simulink model "FOC"  (R2026a)
settings: Solver=FixedStepDiscrete  StopTime=inf  FixedStep=Ts  EnableMultiTasking=on
InitFcn:
  | ParameterInit
undefined symbols (not defined in the file): drive, FAKF, motor, Ts
libraries: mcbhdlcontrolslib x9, matrix_library x8, simulink x7, mcbcontrolslib x5, mcbsensorlessestimatorlib x2, mcbeeMathTransformLib x2, slpidlib x2, mcbpositiondecoderlib x1, sl_discontinuities x1
(part 2 of 2)

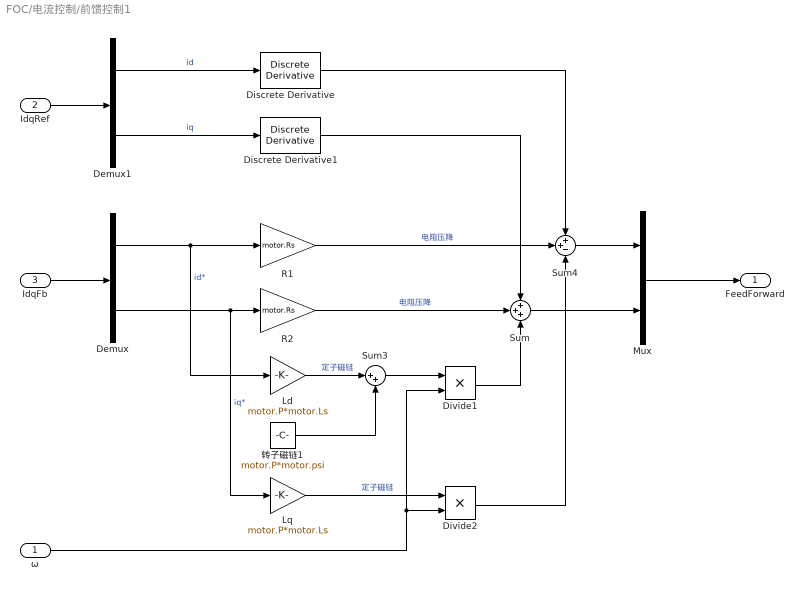
== system FOC/电流控制/前馈控制1 ==
  ω : Inport
  IdqRef : Inport  Port=2
  IdqFb : Inport  Port=3
  Demux : Demux  Outputs=2
  Demux1 : Demux  Outputs=2
  Discrete Derivative : simulink/Discrete/Discrete Derivative  gainval=motor.Ls  ICPrevScaledInput=0.0  OutMin=[]  OutMax=[]  OutDataType=fixdt(1, 16)  OutScaling=2^-10  DoSatur=off
  Discrete Derivative1 : simulink/Discrete/Discrete Derivative  gainval=motor.Ls  ICPrevScaledInput=0.0  OutMin=[]  OutMax=[]  OutDataType=fixdt(1, 16)  OutScaling=2^-10  DoSatur=off
  Divide1 : Product  Inputs=**
  Divide2 : Product  Inputs=**
  Ld : Gain  Gain=motor.P*motor.Ls
  Lq : Gain  Gain=motor.P*motor.Ls
  Mux : Mux  Inputs=2
  R1 : Gain  Gain=motor.Rs
  R2 : Gain  Gain=motor.Rs
  Sum : Sum  Inputs=+++
  Sum3 : Sum  Inputs=|++
  Sum4 : Sum  Inputs=++-
  转子磁链1 : Constant  Value=motor.P*motor.psi  VectorParams1D=off  OutDataTypeStr=single
  FeedForward : Outport
  wires:
  Ld/1 -> Sum3/1  "定子磁链"
  转子磁链1/1 -> Sum3/2
  Lq/1 -> Divide2/1  "定子磁链"
  Sum3/1 -> Divide1/1
  ω/1 -> Divide2/2, Divide1/2
  Demux/1 -> R1/1, Ld/1  "id*"
  Demux/2 -> Lq/1, R2/1  "iq*"
  IdqFb/1 -> Demux/1
  Divide2/1 -> Sum4/3
  Divide1/1 -> Sum/3
  Sum/1 -> Mux/2
  Sum4/1 -> Mux/1
  IdqRef/1 -> Demux1/1
  Demux1/2 -> Discrete Derivative1/1  "iq"
  R2/1 -> Sum/2  "电阻压降"
  R1/1 -> Sum4/2  "电阻压降"
  Discrete Derivative1/1 -> Sum/1
  Discrete Derivative/1 -> Sum4/1
  Mux/1 -> FeedForward/1
  Demux1/1 -> Discrete Derivative/1  "id"

== system FOC/电流控制/电压限幅 ==
  dq_in : Inport
  Limit : Inport  Port=2
  Divide1 : Product  Inputs=*/*
  Math Function1 : Math  Operator=square
  Relational Operator : RelationalOperator  Operator=>  OutDataTypeStr=boolean  RndMeth=Simplest  InputSameDT=off
  Sqrt : Sqrt
  Sum of Elements1 : Sum  Inputs=+
  Switch : Switch  Criteria=u2 > Threshold  SaturateOnIntegerOverflow=off  InputSameDT=off
  dq_out : Outport
  wires:
  Divide1/1 -> Switch/1
  Relational Operator/1 -> Switch/2
  Math Function1/1 -> Sum of Elements1/1
  Switch/1 -> dq_out/1
  Sum of Elements1/1 -> Sqrt/1
  Sqrt/1 -> Relational Operator/1, Divide1/2
  Limit/1 -> Relational Operator/2, Divide1/1
  dq_in/1 -> Divide1/3, Switch/3, Math Function1/1

== system FOC/电流控制/非线性补偿 ==
  U_dq : Inport
  Gain1 : Gain  Gain=[1/(motor.Rs+motor.Ls/Ts) 1/(motor.Rs+motor.Ls/Ts)]
  I_dq : Outport
  wires:
  U_dq/1 -> Gain1/1
  Gain1/1 -> I_dq/1

== system FOC/Observer/AKF/协方差估计 ==
  e~ : Inport
  e^ : Inport  Port=2
  S : Inport  Port=3
  T : Inport  Port=4
  Display : Display
  Display1 : Display
  Unit Delay1 : UnitDelay  InitialCondition=eye(2)  SampleTime=-1
  Unit Delay2 : UnitDelay  InitialCondition=eye(2)  SampleTime=-1
  乘法积分器 : Subsystem
  乘法积分器1 : Subsystem
  息差估计 : Subsystem
  残差估计 : Subsystem
  R : Outport
  Q : Outport  Port=2
  wires:
  Unit Delay2/1 -> 乘法积分器1/2(T)
  T/1 -> Unit Delay2/1
  乘法积分器/1(Q) -> Q/1, Display/1
  乘法积分器1/1(R) -> R/1, Display1/1
  Unit Delay1/1 -> 乘法积分器/2(S)
  息差估计/1(cov) -> 乘法积分器1/1(T~)
  S/1 -> Unit Delay1/1
  e^/1 -> 残差估计/1(ωθ)
  残差估计/1(cov) -> 乘法积分器/1(S~)
  e~/1 -> 息差估计/1(ωθ)

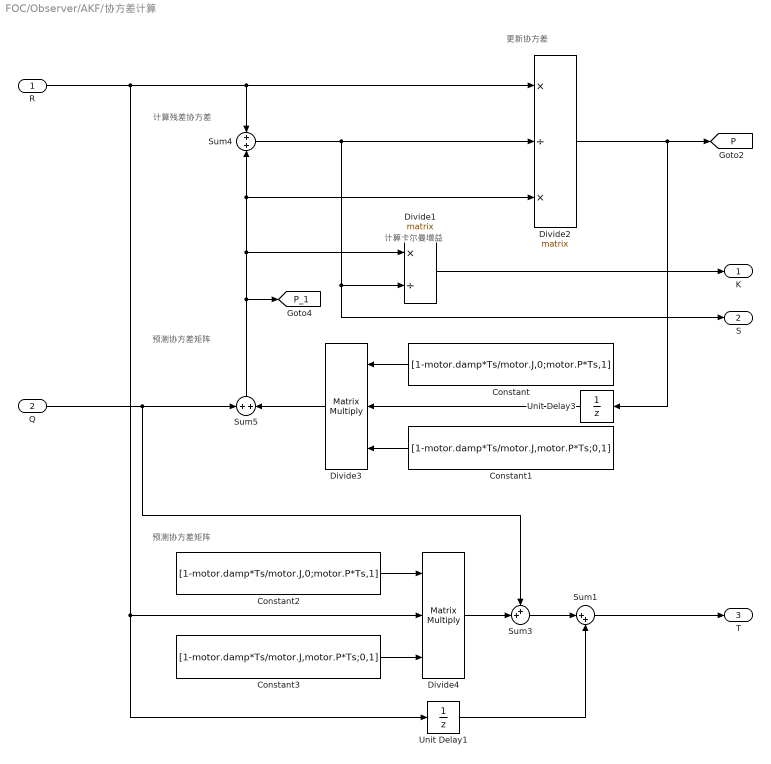
== system FOC/Observer/AKF/协方差计算 ==
  note: 预测协方差矩阵
  note: 更新协方差
  note: 计算卡尔曼增益
  note: 计算残差协方差
  note: 预测协方差矩阵
  R : Inport
  Q : Inport  Port=2
  Constant : Constant  Value=[1-motor.damp*Ts/motor.J,0;motor.P*Ts,1]  VectorParams1D=off  OutDataTypeStr=single
  Constant1 : Constant  Value=[1-motor.damp*Ts/motor.J,motor.P*Ts;0,1]  VectorParams1D=off  OutDataTypeStr=single
  Constant2 : Constant  Value=[1-motor.damp*Ts/motor.J,0;motor.P*Ts,1]  VectorParams1D=off  OutDataTypeStr=single
  Constant3 : Constant  Value=[1-motor.damp*Ts/motor.J,motor.P*Ts;0,1]  VectorParams1D=off  OutDataTypeStr=single
  Divide1 : Product  Inputs=*/  Multiplication=Matrix(*)
  Divide2 : Product  Inputs=*/*  Multiplication=Matrix(*)
  Divide3 : Product  Inputs=***  Multiplication=Matrix(*)
  Divide4 : Product  Inputs=***  Multiplication=Matrix(*)
  Sum1 : Sum  Inputs=|++
  Sum3 : Sum  Inputs=++|
  Sum4 : Sum  Inputs=+|+
  Sum5 : Sum  Inputs=+|+
  Unit Delay1 : UnitDelay  InitialCondition=eye(2)  SampleTime=-1
  Unit Delay3 : UnitDelay  InitialCondition=eye(2)  SampleTime=-1
  K : Outport
  S : Outport  Port=2
  T : Outport  Port=3
  tag scope: P=global, P_1=global
  wires:
  Q/1 -> Sum5/1, Sum3/1
  Unit Delay1/1 -> Sum1/2
  Sum1/1 -> T/1
  R/1 -> Sum4/1, Divide2/1, Divide4/2, Unit Delay1/1
  Sum3/1 -> Sum1/1
  Divide4/1 -> Sum3/2
  Constant2/1 -> Divide4/1
  Constant3/1 -> Divide4/3
  Divide1/1 -> K/1
  Sum4/1 -> Divide2/2, Divide1/2, S/1
  Unit Delay3/1 -> Divide3/2
  Constant1/1 -> Divide3/3
  Divide3/1 -> Sum5/2
  Divide2/1 -> Unit Delay3/1, [P]
  Constant/1 -> Divide3/1
  Sum5/1 -> Sum4/2, Divide2/3, Divide1/1, [P_1]

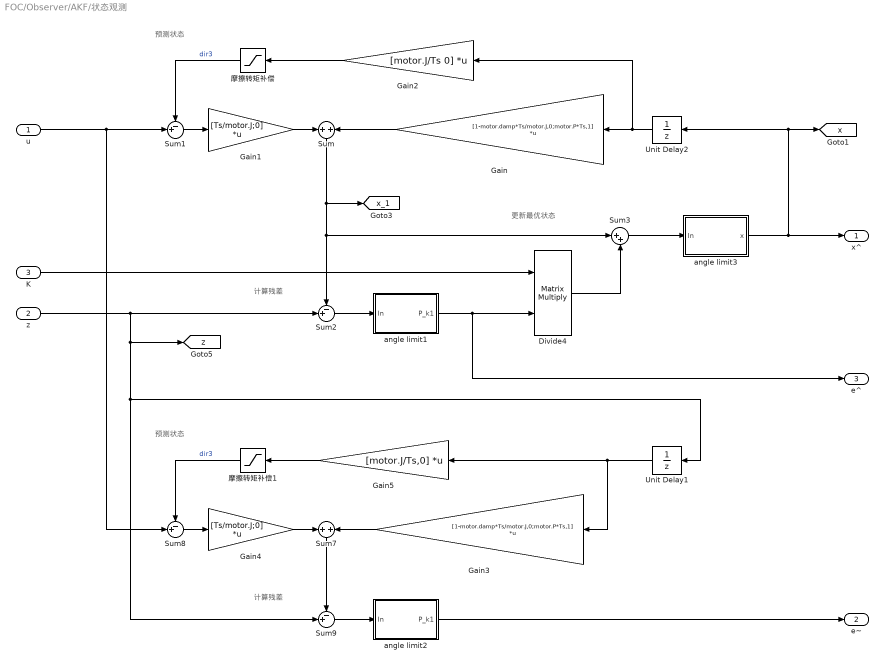
== system FOC/Observer/AKF/状态观测 ==
  note: 计算残差
  note: 预测状态
  note: 更新最优状态
  note: 计算残差
  note: 预测状态
  u : Inport
  z : Inport  Port=2
  K : Inport  Port=3
  Divide4 : Product  Inputs=**  Multiplication=Matrix(*)
  Gain : Gain  Gain=[1-motor.damp*Ts/motor.J,0;motor.P*Ts,1]  Multiplication=Matrix(K*u)
  Gain1 : Gain  Gain=[Ts/motor.J;0]  Multiplication=Matrix(K*u)
  Gain2 : Gain  Gain=[motor.J/Ts 0]  Multiplication=Matrix(K*u)
  Gain3 : Gain  Gain=[1-motor.damp*Ts/motor.J,0;motor.P*Ts,1]  Multiplication=Matrix(K*u)
  Gain4 : Gain  Gain=[Ts/motor.J;0]  Multiplication=Matrix(K*u)
  Gain5 : Gain  Gain=[motor.J/Ts,0]  Multiplication=Matrix(K*u)
  Sum : Sum  Inputs=+|+
  Sum{1..2,8..9} (4 alike) : Sum  Inputs=-+|
  Sum3 : Sum  Inputs=|++
  Sum7 : Sum  Inputs=+|+
  Unit Delay1 : UnitDelay  SampleTime=-1
  Unit Delay2 : UnitDelay  SampleTime=-1
  angle limit1 : Subsystem
  angle limit2 : Subsystem
  angle limit3 : Subsystem
  摩擦转矩补偿 : Saturate  UpperLimit=motor.fric  LowerLimit=-motor.fric
  摩擦转矩补偿1 : Saturate  UpperLimit=motor.fric  LowerLimit=-motor.fric
  x^ : Outport
  e~ : Outport  Port=2
  e^ : Outport  Port=3
  tag scope: x=global, x_1=global, z=global
  wires:
  摩擦转矩补偿/1 -> Sum1/1  "dir3"
  摩擦转矩补偿1/1 -> Sum8/1  "dir3"
  angle limit2/1(P_k1) -> e~/1
  K/1 -> Divide4/1
  z/1 -> Unit Delay1/1, Sum9/2, [z], Sum2/2
  u/1 -> Sum8/2, Sum1/2
  Unit Delay1/1 -> Gain5/1, Gain3/1
  Sum8/1 -> Gain4/1
  Sum2/1 -> angle limit1/1(In)
  Sum9/1 -> angle limit2/1(In)
  angle limit3/1(x) -> Unit Delay2/1, [x], x^/1
  Sum7/1 -> Sum9/1
  Gain2/1 -> 摩擦转矩补偿/1
  Sum1/1 -> Gain1/1
  Divide4/1 -> Sum3/2
  Unit Delay2/1 -> Gain/1, Gain2/1
  Gain5/1 -> 摩擦转矩补偿1/1
  Gain3/1 -> Sum7/2
  Gain/1 -> Sum/2
  Gain1/1 -> Sum/1
  Gain4/1 -> Sum7/1
  Sum3/1 -> angle limit3/1(In)
  angle limit1/1(P_k1) -> Divide4/2, e^/1
  Sum/1 -> Sum3/1, Sum2/1, [x_1]

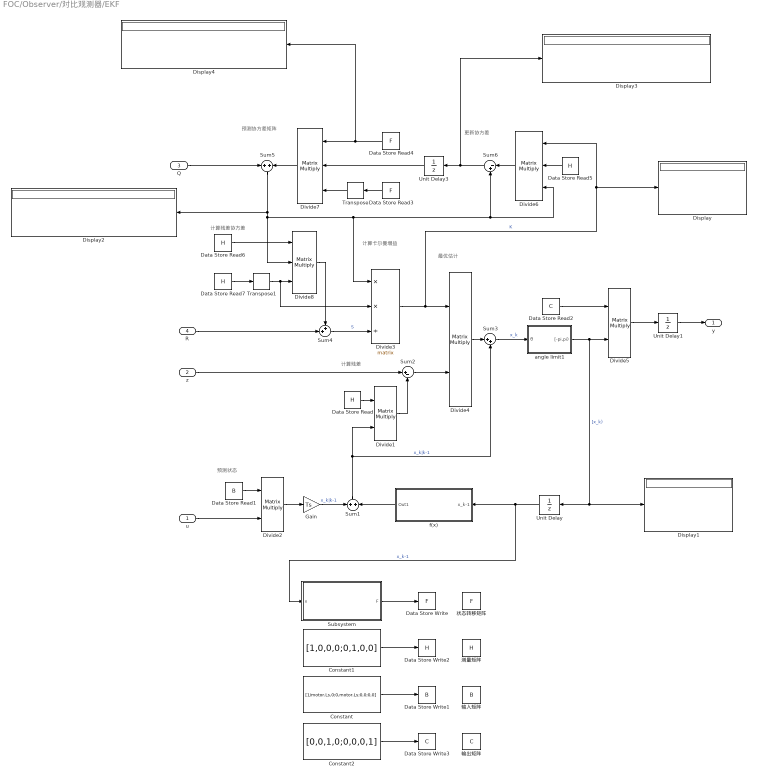
== system FOC/Observer/对比观测器/EKF ==
  note: 更新协方差
  note: 计算卡尔曼增益
  note: 预测协方差矩阵
  note: 计算残差协方差
  note: 最优估计
  note: 计算残差
  note: 预测状态
  u : Inport
  z : Inport  Port=2
  Q : Inport  Port=3
  R : Inport  Port=4
  Constant : Constant  Value=[1/motor.Ls,0;0,motor.Ls;0,0;0,0]  VectorParams1D=off  OutDataTypeStr=single
  Constant1 : Constant  Value=[1,0,0,0;0,1,0,0]  VectorParams1D=off  OutDataTypeStr=single
  Constant2 : Constant  Value=[0,0,1,0;0,0,0,1]  VectorParams1D=off  OutDataTypeStr=single
  Data Store Read{,5..7} (4 alike) : DataStoreRead  DataStoreName=H  IndexOptions=Index vector (dialog)  Indices=1  OutputSizes=1
  Data Store Read1 : DataStoreRead  DataStoreName=B  IndexOptions=Index vector (dialog)  Indices=1  OutputSizes=1
  Data Store Read2 : DataStoreRead  DataStoreName=C  IndexOptions=Index vector (dialog)  Indices=1  OutputSizes=1
  Data Store Read3 : DataStoreRead  DataStoreName=F  IndexOptions=Index vector (dialog)  Indices=1  OutputSizes=1
  Data Store Read4 : DataStoreRead  DataStoreName=F  IndexOptions=Index vector (dialog)  Indices=1  OutputSizes=1
  Data Store Write : DataStoreWrite  DataStoreName=F  IndexOptions=Index vector (dialog)  Indices=1  OutputSizes=1
  Data Store Write1 : DataStoreWrite  DataStoreName=B  IndexOptions=Index vector (dialog)  Indices=1  OutputSizes=1
  Data Store Write2 : DataStoreWrite  DataStoreName=H  IndexOptions=Index vector (dialog)  Indices=1  OutputSizes=1
  Data Store Write3 : DataStoreWrite  DataStoreName=C  IndexOptions=Index vector (dialog)  Indices=1  OutputSizes=1
  Display{,1..4} (5 alike) : Display
  Divide{1..2,4..5} (4 alike) : Product  Inputs=**  Multiplication=Matrix(*)
  Divide3 : Product  Inputs=**/  Multiplication=Matrix(*)
  Divide6 : Product  Inputs=***  Multiplication=Matrix(*)
  Divide7 : Product  Inputs=***  Multiplication=Matrix(*)
  Divide8 : Product  Inputs=***  Multiplication=Matrix(*)
  Gain : Gain  Gain=Ts
  Subsystem : Subsystem
  Sum1 : Sum  Inputs=+|+
  Sum2 : Sum  Inputs=|+-
  Sum3 : Sum  Inputs=|++
  Sum4 : Sum  Inputs=++|
  Sum5 : Sum  Inputs=+|+
  Sum6 : Sum  Inputs=|-+
  Transpose : matrix_library/Transpose
  Transpose1 : matrix_library/Transpose
  Unit Delay : UnitDelay  InitialCondition=zeros(4,1)  SampleTime=-1
  Unit Delay1 : UnitDelay  InitialCondition=zeros(2,1)  SampleTime=-1
  Unit Delay3 : UnitDelay  InitialCondition=diag([1e0,1e0,1000*[1,Ts^2/4]])  SampleTime=-1
  angle limit1 : Subsystem
  f(x) : Subsystem
  测量矩阵 : DataStoreMemory  DataStoreName=H  WriteAfterWriteMsg=warning  InitialValue=[1,0,0,0;0,1,0,0]  VectorParams1D=off  ShowAdditionalParam=off
  状态转移矩阵 : DataStoreMemory  DataStoreName=F  WriteAfterWriteMsg=warning  InitialValue=eye(4)  VectorParams1D=off  ShowAdditionalParam=off
  输入矩阵 : DataStoreMemory  DataStoreName=B  WriteAfterWriteMsg=warning  InitialValue=[1/motor.Ls,0;0,motor.Ls;0,0;0,0]  VectorParams1D=off  ShowAdditionalParam=off
  输出矩阵 : DataStoreMemory  DataStoreName=C  WriteAfterWriteMsg=warning  InitialValue=[0,0,1,0;0,0,0,1]  VectorParams1D=off  ShowAdditionalParam=off
  y : Outport
  wires:
  Data Store Read4/1 -> Divide7/1, Display4/1
  Sum6/1 -> Unit Delay3/1, Display3/1
  Unit Delay1/1 -> y/1
  Divide8/1 -> Sum4/1
  Data Store Read6/1 -> Divide8/1
  Transpose1/1 -> Divide8/3, Divide3/2
  Data Store Read7/1 -> Transpose1/1
  Constant2/1 -> Data Store Write3/1
  Divide1/1 -> Sum2/2
  Data Store Read/1 -> Divide1/1
  Gain/1 -> Sum1/1  "x_k|k-1"
  angle limit1/1("[-pi,pi)") -> Unit Delay/1, Display1/1, Divide5/2  "[x_k)"
  f(x)/1(Out1) -> Sum1/2
  Subsystem/1(F) -> Data Store Write/1
  Transpose/1 -> Divide7/3
  Divide6/1 -> Sum6/1
  Data Store Read5/1 -> Divide6/2
  Data Store Read3/1 -> Transpose/1
  Sum4/1 -> Divide3/3  "S"
  Unit Delay3/1 -> Divide7/2
  R/1 -> Sum4/2
  Divide7/1 -> Sum5/2
  Sum5/1 -> Display2/1, Divide8/2, Sum6/2, Divide6/3, Divide3/1
  Q/1 -> Sum5/1
  Constant1/1 -> Data Store Write2/1
  Constant/1 -> Data Store Write1/1
  Divide5/1 -> Unit Delay1/1
  Data Store Read1/1 -> Divide2/1
  z/1 -> Sum2/1
  Sum2/1 -> Divide4/2
  Divide4/1 -> Sum3/1
  Divide2/1 -> Gain/1
  Unit Delay/1 -> f(x)/1(x_k-1), Subsystem/1(x)  "x_k-1"
  Data Store Read2/1 -> Divide5/1
  u/1 -> Divide2/2
  Sum1/1 -> Sum3/2, Divide1/2  "x_k|k-1"
  Divide3/1 -> Divide4/1, Divide6/1, Display/1  "K"
  Sum3/1 -> angle limit1/1(θ)  "x_k"

== system FOC/Observer/对比观测器/FKF ==
  z : Inport
  u : Inport  Port=2
  AKF : Subsystem
  Demux : Demux  Outputs=2
  位置提取 : Subsystem
  角度转换 : Subsystem
  计算转子反电动势 : Subsystem
  转矩计算 : Subsystem
  ω_m : Outport
  θ_e : Outport  Port=2
  wires:
  位置提取/1(ωθ) -> AKF/2(z_k)  "ωθ~"
  角度转换/1(sincos) -> 位置提取/2(θ_sincos), 转矩计算/1(θ_sincos)
  AKF/1(x_k) -> Demux/1
  u/1 -> 计算转子反电动势/2(Uαβ)
  Demux/1 -> ω_m/1
  Demux/2 -> 角度转换/1(θ), θ_e/1
  计算转子反电动势/1(Eαβ) -> 位置提取/1(Eαβ)  "E_αβ"
  z/1 -> 转矩计算/2(I_αβ), 计算转子反电动势/1(Iαβ)
  转矩计算/1(T) -> AKF/1(u_k)  "T"

== system FOC/Observer/对比观测器/Subsystem ==
  θ_e : Inport
  Constant2 : Constant  Value=-pi  OutDataTypeStr=single
  Constant4 : Constant  Value=pi  OutDataTypeStr=single
  Difference : simulink/Discrete/Difference  ICPrevInput=0.0  OutMin=[]  OutMax=[]  OutDataType=fixdt(1, 16)  OutScaling=2^-10  DoSatur=off
  Gain : Gain  Gain=1/(motor.P*Ts)
  Gain6 : Gain  Gain=-2*pi  OutDataTypeStr=single
  Gain7 : Gain  Gain=2*pi  OutDataTypeStr=single
  Relational Operator2 : RelationalOperator  Operator=<  RndMeth=Simplest  InputSameDT=off
  Relational Operator3 : RelationalOperator  Operator=<=  RndMeth=Simplest  InputSameDT=off
  Sum3 : Sum  Inputs=+++
  Y : Outport
  wires:
  Gain/1 -> Y/1
  Constant2/1 -> Relational Operator2/2
  Relational Operator3/1 -> Gain6/1
  Gain7/1 -> Sum3/3
  Constant4/1 -> Relational Operator3/1
  Relational Operator2/1 -> Gain7/1
  Gain6/1 -> Sum3/1
  Difference/1 -> Relational Operator3/2, Sum3/2, Relational Operator2/1
  Sum3/1 -> Gain/1
  θ_e/1 -> Difference/1

== system FOC/Observer/对比观测器/Subsystem1 ==
  0-2pi : Inport
  Constant3 : Constant  Value=-pi  OutDataTypeStr=single
  Constant4 : Constant  Value=pi  OutDataTypeStr=single
  Gain6 : Gain  Gain=-2*pi  OutDataTypeStr=single
  Gain7 : Gain  Gain=2*pi  OutDataTypeStr=single
  Relational Operator2 : RelationalOperator  Operator=<  RndMeth=Simplest  InputSameDT=off
  Relational Operator3 : RelationalOperator  Operator=<  RndMeth=Simplest  InputSameDT=off
  Sum3 : Sum  Inputs=+++
  -pi-pi : Outport
  wires:
  Sum3/1 -> -pi-pi/1
  Gain7/1 -> Sum3/3
  Gain6/1 -> Sum3/1
  Relational Operator3/1 -> Gain6/1
  Relational Operator2/1 -> Gain7/1
  0-2pi/1 -> Relational Operator3/2, Sum3/2, Relational Operator2/1
  Constant3/1 -> Relational Operator2/2
  Constant4/1 -> Relational Operator3/1

== system FOC/Observer/对比观测器/Subsystem2 ==
  0-2pi : Inport
  Constant3 : Constant  Value=-pi  OutDataTypeStr=single
  Constant4 : Constant  Value=pi  OutDataTypeStr=single
  Gain6 : Gain  Gain=-2*pi  OutDataTypeStr=single
  Gain7 : Gain  Gain=2*pi  OutDataTypeStr=single
  Relational Operator2 : RelationalOperator  Operator=<  RndMeth=Simplest  InputSameDT=off
  Relational Operator3 : RelationalOperator  Operator=<  RndMeth=Simplest  InputSameDT=off
  Sum3 : Sum  Inputs=+++
  -pi-pi : Outport
  wires:
  Constant4/1 -> Relational Operator3/1
  Constant3/1 -> Relational Operator2/2
  0-2pi/1 -> Relational Operator2/1, Sum3/2, Relational Operator3/2
  Relational Operator2/1 -> Gain7/1
  Relational Operator3/1 -> Gain6/1
  Gain6/1 -> Sum3/1
  Gain7/1 -> Sum3/3
  Sum3/1 -> -pi-pi/1

== system FOC/Observer/对比观测器/Subsystem3 ==
  0-2pi : Inport
  Constant3 : Constant  Value=-pi  OutDataTypeStr=single
  Constant4 : Constant  Value=pi  OutDataTypeStr=single
  Gain6 : Gain  Gain=-2*pi  OutDataTypeStr=single
  Gain7 : Gain  Gain=2*pi  OutDataTypeStr=single
  Relational Operator2 : RelationalOperator  Operator=<  RndMeth=Simplest  InputSameDT=off
  Relational Operator3 : RelationalOperator  Operator=<  RndMeth=Simplest  InputSameDT=off
  Sum3 : Sum  Inputs=+++
  -pi-pi : Outport
  wires:
  Sum3/1 -> -pi-pi/1
  Gain7/1 -> Sum3/3
  Gain6/1 -> Sum3/1
  Relational Operator3/1 -> Gain6/1
  Relational Operator2/1 -> Gain7/1
  0-2pi/1 -> Relational Operator3/2, Sum3/2, Relational Operator2/1
  Constant3/1 -> Relational Operator2/2
  Constant4/1 -> Relational Operator3/1

== system FOC/Observer/AKF/协方差估计/乘法积分器 ==
  note: 矩阵指数运算量比较大，用一阶泰勒展开式近似
  S~ : Inport
  S : Inport  Port=2
  Divide1 : Product  Inputs=*/  Multiplication=Matrix(*)
  Divide2 : Product  Inputs=***  Multiplication=Matrix(*)
  Gain1 : Gain  Gain=FAKF.fg
  Gain2 : Gain  Gain=1-FAKF.fg
  Sum3 : Sum  Inputs=|++
  Transpose2 : matrix_library/Transpose
  Unit Delay2 : UnitDelay  InitialCondition=eye(2)  SampleTime=-1
  Q : Outport
  wires:
  S/1 -> Divide1/2
  S~/1 -> Divide1/1
  Sum3/1 -> Q/1, Unit Delay2/1
  Transpose2/1 -> Divide2/3
  Gain1/1 -> Sum3/1
  Divide1/1 -> Transpose2/1, Divide2/1
  Gain2/1 -> Sum3/2
  Divide2/1 -> Gain1/1
  Unit Delay2/1 -> Gain2/1, Divide2/2

== system FOC/Observer/AKF/协方差估计/乘法积分器1 ==
  note: 矩阵指数运算量比较大，用一阶泰勒展开式近似
  T~ : Inport
  T : Inport  Port=2
  Divide1 : Product  Inputs=*/  Multiplication=Matrix(*)
  Divide2 : Product  Inputs=***  Multiplication=Matrix(*)
  Gain1 : Gain  Gain=FAKF.fg
  Gain2 : Gain  Gain=1-FAKF.fg
  Sum3 : Sum  Inputs=|++
  Transpose2 : matrix_library/Transpose
  Unit Delay2 : UnitDelay  InitialCondition=eye(2)  SampleTime=-1
  R : Outport
  wires:
  Unit Delay2/1 -> Divide2/2, Gain2/1
  Divide2/1 -> Gain1/1
  Gain2/1 -> Sum3/2
  Divide1/1 -> Divide2/1, Transpose2/1
  Gain1/1 -> Sum3/1
  Transpose2/1 -> Divide2/3
  Sum3/1 -> Unit Delay2/1, R/1
  T~/1 -> Divide1/1
  T/1 -> Divide1/2

== system FOC/Observer/AKF/协方差估计/息差估计 ==
  ωθ : Inport
  Demux1 : Demux  Outputs=2
  IIR Filter1 : mcbcontrolslib/IIR Filter  VariantControl=Low Pass Filter  VariantSelect=Low-pass  FilterConstantInputType=Specify via dialog  Filter_constant=FAKF.fg  InitialOutput=Specify via dialog  InitialOutputValue=0  ExternalReset=none  advancedSettings=off  Ts=50e-6  cutOff_freq=167.5315
  Matrix Concatenate : Concatenate  Mode=Multidimensional array
  Matrix Concatenate1 : Concatenate  Mode=Multidimensional array
  Matrix Concatenate2 : Concatenate  Mode=Multidimensional array  ConcatenateDimension=2
  Product : Product
  Product1 : Product
  Product3 : Product
  cov : Outport
  wires:
  IIR Filter1/1 -> cov/1
  Demux1/2 -> Product1/2, Product3/1, Product3/2
  ωθ/1 -> Demux1/1
  Product3/1 -> Matrix Concatenate1/2
  Product1/1 -> Matrix Concatenate1/1, Matrix Concatenate/2
  Product/1 -> Matrix Concatenate/1
  Matrix Concatenate/1 -> Matrix Concatenate2/1
  Matrix Concatenate1/1 -> Matrix Concatenate2/2
  Matrix Concatenate2/1 -> IIR Filter1/1
  Demux1/1 -> Product/2, Product/1, Product1/1

== system FOC/Observer/AKF/协方差估计/残差估计 ==
  ωθ : Inport
  Demux1 : Demux  Outputs=2
  Gain : Gain  Gain=Ts/2
  IIR Filter1 : mcbcontrolslib/IIR Filter  VariantControl=Low Pass Filter  VariantSelect=Low-pass  FilterConstantInputType=Specify via dialog  Filter_constant=FAKF.fg  InitialOutput=Specify via dialog  InitialOutputValue=0  ExternalReset=none  advancedSettings=off  Ts=50e-6  cutOff_freq=167.5315
  Matrix Concatenate : Concatenate  Mode=Multidimensional array
  Matrix Concatenate1 : Concatenate  Mode=Multidimensional array
  Matrix Concatenate2 : Concatenate  Mode=Multidimensional array  ConcatenateDimension=2
  Product : Product
  Product1 : Product
  Product3 : Product
  cov : Outport
  wires:
  Demux1/1 -> Product1/1, Product/1, Product/2, Gain/1
  IIR Filter1/1 -> cov/1
  Matrix Concatenate2/1 -> IIR Filter1/1
  Matrix Concatenate1/1 -> Matrix Concatenate2/2
  Matrix Concatenate/1 -> Matrix Concatenate2/1
  Product/1 -> Matrix Concatenate/1
  Product1/1 -> Matrix Concatenate/2, Matrix Concatenate1/1
  Product3/1 -> Matrix Concatenate1/2
  ωθ/1 -> Demux1/1
  Gain/1 -> Product3/1, Product3/2, Product1/2

== system FOC/Observer/AKF/状态观测/angle limit1 ==
  In : Inport
  Constant2 : Constant  Value=-pi  OutDataTypeStr=single
  Constant4 : Constant  Value=pi  OutDataTypeStr=single
  Demux : Demux  Outputs=2
  Gain6 : Gain  Gain=-2*pi  OutDataTypeStr=single
  Gain7 : Gain  Gain=2*pi  OutDataTypeStr=single
  Mux : Mux  Inputs=2
  Relational Operator2 : RelationalOperator  Operator=<  RndMeth=Simplest  InputSameDT=off
  Relational Operator3 : RelationalOperator  Operator=<  RndMeth=Simplest  InputSameDT=off
  Sum3 : Sum  Inputs=+++
  P_k1 : Outport
  wires:
  Constant2/1 -> Relational Operator2/2
  Demux/2 -> Relational Operator3/2, Sum3/2, Relational Operator2/1
  Constant4/1 -> Relational Operator3/1
  Relational Operator3/1 -> Gain6/1
  Gain7/1 -> Sum3/3
  Relational Operator2/1 -> Gain7/1
  Gain6/1 -> Sum3/1
  Sum3/1 -> Mux/2
  In/1 -> Demux/1
  Mux/1 -> P_k1/1
  Demux/1 -> Mux/1

== system FOC/Observer/AKF/状态观测/angle limit2 ==
  In : Inport
  Constant2 : Constant  Value=-pi  OutDataTypeStr=single
  Constant4 : Constant  Value=pi  OutDataTypeStr=single
  Demux : Demux  Outputs=2
  Gain6 : Gain  Gain=-2*pi  OutDataTypeStr=single
  Gain7 : Gain  Gain=2*pi  OutDataTypeStr=single
  Mux : Mux  Inputs=2
  Relational Operator2 : RelationalOperator  Operator=<  RndMeth=Simplest  InputSameDT=off
  Relational Operator3 : RelationalOperator  Operator=<  RndMeth=Simplest  InputSameDT=off
  Sum3 : Sum  Inputs=+++
  P_k1 : Outport
  wires:
  Constant2/1 -> Relational Operator2/2
  Demux/2 -> Relational Operator3/2, Sum3/2, Relational Operator2/1
  Constant4/1 -> Relational Operator3/1
  Relational Operator3/1 -> Gain6/1
  Gain7/1 -> Sum3/3
  Relational Operator2/1 -> Gain7/1
  Gain6/1 -> Sum3/1
  Sum3/1 -> Mux/2
  In/1 -> Demux/1
  Mux/1 -> P_k1/1
  Demux/1 -> Mux/1

== system FOC/Observer/AKF/状态观测/angle limit3 ==
  In : Inport
  Constant2 : Constant  Value=-pi  OutDataTypeStr=single
  Constant4 : Constant  Value=pi  OutDataTypeStr=single
  Demux : Demux  Outputs=2
  Gain6 : Gain  Gain=-2*pi  OutDataTypeStr=single
  Gain7 : Gain  Gain=2*pi  OutDataTypeStr=single
  Mux : Mux  Inputs=2
  Relational Operator2 : RelationalOperator  Operator=<  RndMeth=Simplest  InputSameDT=off
  Relational Operator3 : RelationalOperator  Operator=<  RndMeth=Simplest  InputSameDT=off
  Sum3 : Sum  Inputs=+++
  x : Outport
  wires:
  Demux/1 -> Mux/1
  Mux/1 -> x/1
  In/1 -> Demux/1
  Sum3/1 -> Mux/2
  Gain6/1 -> Sum3/1
  Relational Operator2/1 -> Gain7/1
  Gain7/1 -> Sum3/3
  Relational Operator3/1 -> Gain6/1
  Constant4/1 -> Relational Operator3/1
  Demux/2 -> Relational Operator2/1, Sum3/2, Relational Operator3/2
  Constant2/1 -> Relational Operator2/2

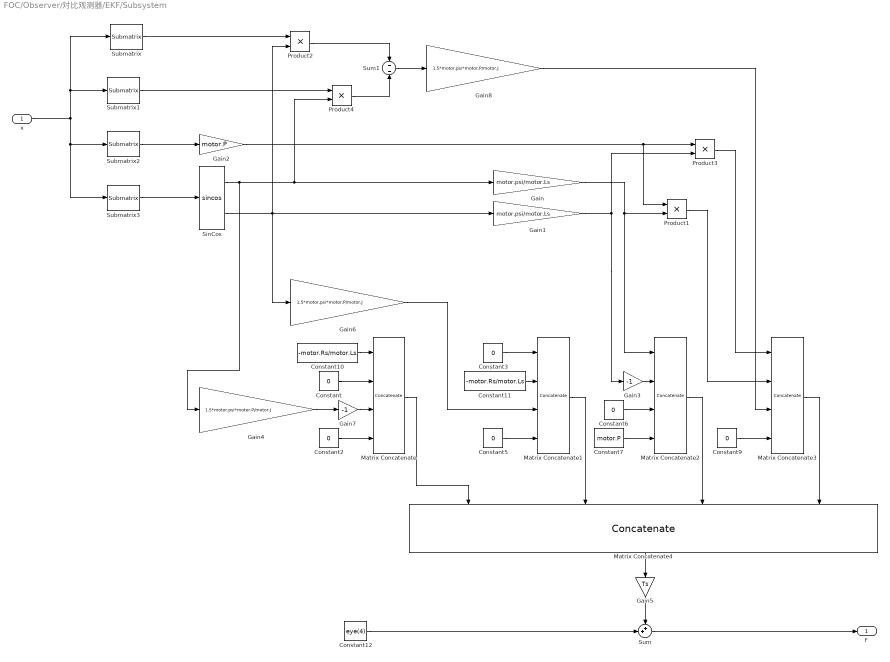
== system FOC/Observer/对比观测器/EKF/Subsystem ==
  x : Inport
  Constant{,2..3,5..6,9} (6 alike) : Constant  Value=0  OutDataTypeStr=single
  Constant10 : Constant  Value=-motor.Rs/motor.Ls  OutDataTypeStr=single
  Constant11 : Constant  Value=-motor.Rs/motor.Ls  OutDataTypeStr=single
  Constant12 : Constant  Value=eye(4)  OutDataTypeStr=single
  Constant7 : Constant  Value=motor.P  OutDataTypeStr=single
  Gain : Gain  Gain=motor.psi/motor.Ls
  Gain1 : Gain  Gain=motor.psi/motor.Ls
  Gain2 : Gain  Gain=motor.P
  Gain3 : Gain  Gain=-1
  Gain4 : Gain  Gain=1.5*motor.psi*motor.P/motor.J
  Gain5 : Gain  Gain=Ts
  Gain6 : Gain  Gain=1.5*motor.psi*motor.P/motor.J
  Gain7 : Gain  Gain=-1
  Gain8 : Gain  Gain=1.5*motor.psi*motor.P/motor.J
  Matrix Concatenate{,1..3} (4 alike) : Concatenate  NumInputs=4  Mode=Multidimensional array
  Matrix Concatenate4 : Concatenate  NumInputs=4  Mode=Multidimensional array  ConcatenateDimension=2
  Product{1..4} (4 alike) : Product
  SinCos : Trigonometry  Operator=sincos
  Submatrix : matrix_library/Submatrix  RowSpan=Range of rows  RowStartMode=Index  RowStartIndex=1  RowEndMode=Index  RowEndIndex=1  ColSpan=One column  ColStartMode=First  ColStartIndex=1  ColEndMode=Index  ColEndIndex=1
  Submatrix1 : matrix_library/Submatrix  RowSpan=Range of rows  RowStartMode=Index  RowStartIndex=2  RowEndMode=Index  RowEndIndex=2  ColSpan=One column  ColStartMode=First  ColStartIndex=1  ColEndMode=Index  ColEndIndex=1
  Submatrix2 : matrix_library/Submatrix  RowSpan=Range of rows  RowStartMode=Index  RowStartIndex=3  RowEndMode=Index  RowEndIndex=3  ColSpan=One column  ColStartMode=First  ColStartIndex=1  ColEndMode=Index  ColEndIndex=1
  Submatrix3 : matrix_library/Submatrix  RowSpan=Range of rows  RowStartMode=Index  RowStartIndex=4  RowEndMode=Index  RowEndIndex=4  ColSpan=One column  ColStartMode=First  ColStartIndex=1  ColEndMode=Index  ColEndIndex=1
  Sum : Sum  Inputs=++|
  Sum1 : Sum  Inputs=-|-
  F : Outport
  wires:
  Sum1/1 -> Gain8/1
  Product4/1 -> Sum1/2
  Product2/1 -> Sum1/1
  Submatrix1/1 -> Product4/1
  Submatrix/1 -> Product2/1
  Gain7/1 -> Matrix Concatenate/3
  Gain3/1 -> Matrix Concatenate2/2
  Gain2/1 -> Product3/1, Product1/1
  Submatrix2/1 -> Gain2/1
  Submatrix3/1 -> SinCos/1
  Gain5/1 -> Sum/1
  Matrix Concatenate4/1 -> Gain5/1
  Constant12/1 -> Sum/2
  Gain1/1 -> Gain3/1, Product3/2
  SinCos/2 -> Gain1/1, Product2/2, Gain6/1
  SinCos/1 -> Gain4/1, Product4/2, Gain/1
  x/1 -> Submatrix/1, Submatrix1/1, Submatrix2/1, Submatrix3/1
  Product1/1 -> Matrix Concatenate3/2
  Product3/1 -> Matrix Concatenate3/1
  Gain/1 -> Product1/2, Matrix Concatenate2/1
  Matrix Concatenate3/1 -> Matrix Concatenate4/4
  Constant9/1 -> Matrix Concatenate3/4
  Constant11/1 -> Matrix Concatenate1/2
  Matrix Concatenate2/1 -> Matrix Concatenate4/3
  Gain4/1 -> Gain7/1
  Matrix Concatenate1/1 -> Matrix Concatenate4/2
  Gain6/1 -> Matrix Concatenate1/3
  Gain8/1 -> Matrix Concatenate3/3
  Constant10/1 -> Matrix Concatenate/1
  Constant6/1 -> Matrix Concatenate2/3
  Sum/1 -> F/1
  Constant7/1 -> Matrix Concatenate2/4
  Matrix Concatenate/1 -> Matrix Concatenate4/1
  Constant5/1 -> Matrix Concatenate1/4
  Constant3/1 -> Matrix Concatenate1/1
  Constant/1 -> Matrix Concatenate/2
  Constant2/1 -> Matrix Concatenate/4

== system FOC/Observer/对比观测器/EKF/angle limit1 ==
  θ : Inport
  Constant2 : Constant  Value=-pi  OutDataTypeStr=single
  Constant4 : Constant  Value=pi  OutDataTypeStr=single
  Demux : Demux
  Gain6 : Gain  Gain=-2*pi  OutDataTypeStr=single
  Gain7 : Gain  Gain=2*pi  OutDataTypeStr=single
  Mux : Mux
  Relational Operator2 : RelationalOperator  Operator=<  RndMeth=Simplest  InputSameDT=off
  Relational Operator3 : RelationalOperator  Operator=<=  RndMeth=Simplest  InputSameDT=off
  Sum3 : Sum  Inputs=+++
  "[-pi,pi)" : Outport
  wires:
  Demux/2 -> Mux/2
  Demux/3 -> Mux/3
  Constant2/1 -> Relational Operator2/2
  Demux/4 -> Relational Operator3/2, Sum3/2, Relational Operator2/1
  Constant4/1 -> Relational Operator3/1
  Relational Operator3/1 -> Gain6/1
  Gain7/1 -> Sum3/3
  Relational Operator2/1 -> Gain7/1
  Gain6/1 -> Sum3/1
  Sum3/1 -> Mux/4
  θ/1 -> Demux/1
  Mux/1 -> "[-pi,pi)"/1
  Demux/1 -> Mux/1

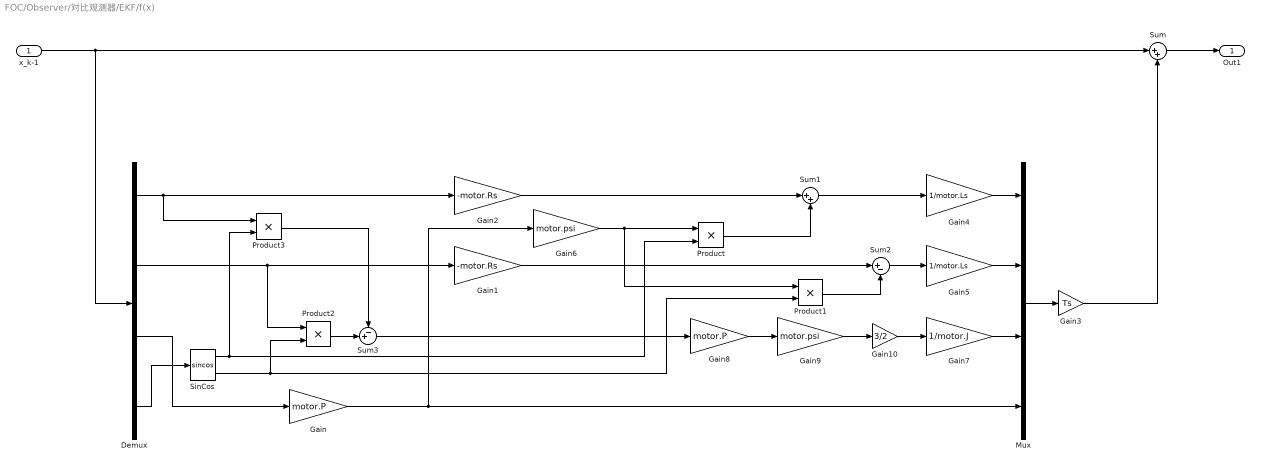
== system FOC/Observer/对比观测器/EKF/f(x) ==
  x_k-1 : Inport
  Demux : Demux
  Gain : Gain  Gain=motor.P
  Gain1 : Gain  Gain=-motor.Rs
  Gain10 : Gain  Gain=3/2
  Gain2 : Gain  Gain=-motor.Rs
  Gain3 : Gain  Gain=Ts
  Gain4 : Gain  Gain=1/motor.Ls
  Gain5 : Gain  Gain=1/motor.Ls
  Gain6 : Gain  Gain=motor.psi
  Gain7 : Gain  Gain=1/motor.J
  Gain8 : Gain  Gain=motor.P
  Gain9 : Gain  Gain=motor.psi
  Mux : Mux
  Product{,1..3} (4 alike) : Product
  SinCos : Trigonometry  Operator=sincos
  Sum : Sum  Inputs=|++
  Sum1 : Sum  Inputs=|++
  Sum2 : Sum  Inputs=|+-
  Sum3 : Sum  Inputs=-+|
  Out1 : Outport
  wires:
  Sum3/1 -> Gain8/1
  Product3/1 -> Sum3/1
  Product2/1 -> Sum3/2
  Gain9/1 -> Gain10/1
  Gain10/1 -> Gain7/1
  Gain8/1 -> Gain9/1
  SinCos/2 -> Product2/2, Product1/2
  Product1/1 -> Sum2/2
  SinCos/1 -> Product3/2, Product/2
  Gain6/1 -> Product/1, Product1/1
  Product/1 -> Sum1/2
  Gain/1 -> Mux/4, Gain6/1
  Sum/1 -> Out1/1
  Demux/3 -> Gain/1
  Gain7/1 -> Mux/3
  Demux/4 -> SinCos/1
  Gain5/1 -> Mux/2
  Gain4/1 -> Mux/1
  Gain3/1 -> Sum/2
  Sum2/1 -> Gain5/1
  Sum1/1 -> Gain4/1
  Gain1/1 -> Sum2/1
  Demux/2 -> Product2/1, Gain1/1
  Gain2/1 -> Sum1/1
  Demux/1 -> Product3/1, Gain2/1
  Mux/1 -> Gain3/1
  x_k-1/1 -> Sum/1, Demux/1

== system FOC/Observer/对比观测器/FKF/AKF ==
  u_k : Inport
  z_k : Inport  Port=2
  Constant1 : Constant  Value=[0.1421,-0.077657;0.0001717,0.002415]  VectorParams1D=off  OutDataTypeStr=single
  Constant4 : Constant  Value=[0.3508,7.253;0.000117,0.0586]  VectorParams1D=off  OutDataTypeStr=single
  状态观测 : Subsystem
  x_k : Outport
  wires:
  Constant4/1 -> 状态观测/3(K)  "K"
  状态观测/1(x^) -> x_k/1  "x^"
  z_k/1 -> 状态观测/2(z)
  u_k/1 -> 状态观测/1(u)

== system FOC/Observer/对比观测器/FKF/位置提取 ==
  Eαβ : Inport
  θ_sincos : Inport  Port=2
  Constant : Constant  Value=motor.psi  OutDataTypeStr=single
  Demux : Demux  Outputs=2
  Divide3 : Product  Inputs=/*
  Gain : Gain  Gain=[-1 1]  Multiplication=Matrix(K*u)
  Gain1 : Gain  Gain=motor.P
  Gain2 : Gain  Gain=-1
  Mux : Mux  Inputs=2
  Product : Product
  Product1 : Product
  Sign : Signum
  Unit Delay : UnitDelay  SampleTime=-1
  幅角 : mcbcontrolslib/atan2  ApproximationMethod=None  NumberOfIterations=11  NumberOfDataPoints=16  InterpMethod=Flat  outputUnit=Radians  TableDataTypeStr=Inherit: Inherit via input
  ωθ : Outport
  wires:
  Product1/1 -> Demux/1
  Sign/1 -> Product1/1
  Eαβ/1 -> Product1/2, Product/2
  Gain2/1 -> 幅角/1
  Demux/1 -> Gain2/1
  Demux/2 -> 幅角/2
  Mux/1 -> ωθ/1
  Divide3/1 -> Mux/1
  Gain/1 -> Sign/1, Divide3/2
  Product/1 -> Gain/1
  Unit Delay/1 -> Product/1
  θ_sincos/1 -> Unit Delay/1
  幅角/1 -> Mux/2
  Gain1/1 -> Divide3/1
  Constant/1 -> Gain1/1

== system FOC/Observer/对比观测器/FKF/角度转换 ==
  θ : Inport
  Mux1 : Mux  Inputs=2
  SinCos : Trigonometry  Operator=sincos
  sincos : Outport
  wires:
  Mux1/1 -> sincos/1
  SinCos/2 -> Mux1/2
  θ/1 -> SinCos/1
  SinCos/1 -> Mux1/1

== system FOC/Observer/对比观测器/FKF/计算转子反电动势 ==
  Iαβ : Inport
  Uαβ : Inport  Port=2
  Sum5 : Sum  Inputs=+--
  滞后补偿 : DiscreteFilter  Numerator=[0 0 1 1]  Denominator=[2 0 0 0]
  电感分压 : simulink/Discrete/Discrete Derivative  gainval=motor.Ls  ICPrevScaledInput=0.0  OutMin=[]  OutMax=[]  OutDataType=fixdt(1, 16)  OutScaling=2^-10  DoSatur=off
  电阻分压 : Gain  Gain=motor.Rs
  Eαβ : Outport
  wires:
  Sum5/1 -> Eαβ/1
  滞后补偿/1 -> Sum5/1
  Iαβ/1 -> 电阻分压/1, 电感分压/1
  Uαβ/1 -> 滞后补偿/1
  电阻分压/1 -> Sum5/2
  电感分压/1 -> Sum5/3

== system FOC/Observer/对比观测器/FKF/转矩计算 ==
  θ_sincos : Inport
  I_αβ : Inport  Port=2
  Constant : Constant  Value=motor.psi  OutDataTypeStr=single
  Divide1 : Product  Inputs=**
  Gain : Gain  Gain=[-1 1]  Multiplication=Matrix(K*u)
  Gain1 : Gain  Gain=motor.P
  Gain2 : Gain  Gain=1.5
  Product3 : Product
  Unit Delay : UnitDelay  SampleTime=-1
  T : Outport
  wires:
  Gain2/1 -> T/1
  Gain1/1 -> Divide1/2
  θ_sincos/1 -> Unit Delay/1
  I_αβ/1 -> Product3/2
  Unit Delay/1 -> Product3/1
  Gain/1 -> Divide1/1
  Divide1/1 -> Gain2/1
  Constant/1 -> Gain1/1
  Product3/1 -> Gain/1

== system FOC/Observer/对比观测器/FKF/AKF/状态观测 ==
  note: 更新最优状态
  note: 计算残差
  note: 预测状态
  u : Inport
  z : Inport  Port=2
  K : Inport  Port=3
  Divide4 : Product  Inputs=**  Multiplication=Matrix(*)
  Gain : Gain  Gain=[1-motor.damp*Ts/motor.J,0;motor.P*Ts,1]  Multiplication=Matrix(K*u)
  Gain1 : Gain  Gain=[Ts/motor.J;0]  Multiplication=Matrix(K*u)
  Gain2 : Gain  Gain=[motor.J/Ts 0]  Multiplication=Matrix(K*u)
  Sum : Sum  Inputs=+|+
  Sum1 : Sum  Inputs=-+|
  Sum2 : Sum  Inputs=-+|
  Sum3 : Sum  Inputs=|++
  Unit Delay2 : UnitDelay  SampleTime=-1
  angle limit1 : Subsystem
  angle limit3 : Subsystem
  摩擦转矩补偿 : Saturate  UpperLimit=motor.fric  LowerLimit=-motor.fric
  x^ : Outport
  wires:
  摩擦转矩补偿/1 -> Sum1/1  "dir3"
  K/1 -> Divide4/1
  z/1 -> Sum2/2
  u/1 -> Sum1/2
  Sum2/1 -> angle limit1/1(In)
  angle limit3/1(x) -> Unit Delay2/1, x^/1
  Gain2/1 -> 摩擦转矩补偿/1
  Sum1/1 -> Gain1/1
  Divide4/1 -> Sum3/2
  Unit Delay2/1 -> Gain/1, Gain2/1
  Gain/1 -> Sum/2
  Gain1/1 -> Sum/1
  Sum3/1 -> angle limit3/1(In)
  angle limit1/1(P_k1) -> Divide4/2
  Sum/1 -> Sum3/1, Sum2/1

== system FOC/Observer/对比观测器/FKF/AKF/状态观测/angle limit1 ==
  In : Inport
  Constant2 : Constant  Value=-pi  OutDataTypeStr=single
  Constant4 : Constant  Value=pi  OutDataTypeStr=single
  Demux : Demux  Outputs=2
  Gain6 : Gain  Gain=-2*pi  OutDataTypeStr=single
  Gain7 : Gain  Gain=2*pi  OutDataTypeStr=single
  Mux : Mux  Inputs=2
  Relational Operator2 : RelationalOperator  Operator=<  RndMeth=Simplest  InputSameDT=off
  Relational Operator3 : RelationalOperator  Operator=<  RndMeth=Simplest  InputSameDT=off
  Sum3 : Sum  Inputs=+++
  P_k1 : Outport
  wires:
  Constant2/1 -> Relational Operator2/2
  Demux/2 -> Relational Operator3/2, Sum3/2, Relational Operator2/1
  Constant4/1 -> Relational Operator3/1
  Relational Operator3/1 -> Gain6/1
  Gain7/1 -> Sum3/3
  Relational Operator2/1 -> Gain7/1
  Gain6/1 -> Sum3/1
  Sum3/1 -> Mux/2
  In/1 -> Demux/1
  Mux/1 -> P_k1/1
  Demux/1 -> Mux/1

== system FOC/Observer/对比观测器/FKF/AKF/状态观测/angle limit3 ==
  In : Inport
  Constant2 : Constant  Value=-pi  OutDataTypeStr=single
  Constant4 : Constant  Value=pi  OutDataTypeStr=single
  Demux : Demux  Outputs=2
  Gain6 : Gain  Gain=-2*pi  OutDataTypeStr=single
  Gain7 : Gain  Gain=2*pi  OutDataTypeStr=single
  Mux : Mux  Inputs=2
  Relational Operator2 : RelationalOperator  Operator=<  RndMeth=Simplest  InputSameDT=off
  Relational Operator3 : RelationalOperator  Operator=<  RndMeth=Simplest  InputSameDT=off
  Sum3 : Sum  Inputs=+++
  x : Outport
  wires:
  Demux/1 -> Mux/1
  Mux/1 -> x/1
  In/1 -> Demux/1
  Sum3/1 -> Mux/2
  Gain6/1 -> Sum3/1
  Relational Operator2/1 -> Gain7/1
  Gain7/1 -> Sum3/3
  Relational Operator3/1 -> Gain6/1
  Constant4/1 -> Relational Operator3/1
  Demux/2 -> Relational Operator2/1, Sum3/2, Relational Operator3/2
  Constant2/1 -> Relational Operator2/2
